simulink model "lecture8_heat"  (Simulink 7.1)
settings: Solver=FixedStepDiscrete  StartTime=0.0  StopTime=Inf  RelTol=1e-3
libraries: simulink x2
settings Model: Creator=pit  LastModifiedBy=pit

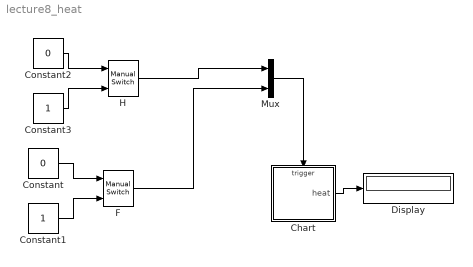
== system lecture8_heat ==
  Chart : Stateflow chart
  Constant : Constant  Value=0  OutDataType=sfix(16)  OutScaling=2^0
  Constant1 : Constant  OutDataType=sfix(16)  OutScaling=2^0
  Constant2 : Constant  Value=0  OutDataType=sfix(16)  OutScaling=2^0
  Constant3 : Constant  OutDataType=sfix(16)  OutScaling=2^0
  Display : Display
  F : simulink/Signal Routing/Manual Switch  SystemSampleTime=-1  sw=1  action=0  varsize=off
  H : simulink/Signal Routing/Manual Switch  SystemSampleTime=-1  sw=0  action=0  varsize=off
  Mux : Mux  Inputs=2
  wires:
  Constant/1 -> F/1
  Constant1/1 -> F/2
  Constant2/1 -> H/1
  Constant3/1 -> H/2
  H/1 -> Mux/1
  F/1 -> Mux/2
  Mux/1 -> Chart/Trigger
  Chart/1(heat) -> Display/1

== stateflow chart Chart ==
  settings: sampleTime=0.1
  state Off
    entry: heat=0
  state H
    entry: heat=0.5
  state F
    entry: heat=1.0
  (default) -> Off
  Off -> H [order 1] : pressH
  Off -> F [order 2] : pressF
  F -> Off [order 1] : pressF
  H -> Off [order 1] : pressH
  H -> F [order 2] : pressF
  F -> H [order 2] : pressH
  data: heat output double
  events: pressH input EITHER_EDGE_EVENT; pressF input EITHER_EDGE_EVENT
